simulink library "discreteClampingPID"  (R2022a)
settings: Solver=VariableStepAuto  StartTime=0.0  StopTime=10.0  RelTol=1e-3
undefined symbols (not defined in the file): Ts
libraries: simulink x4
settings Model: Creator=adabney  LastModifiedBy=maull

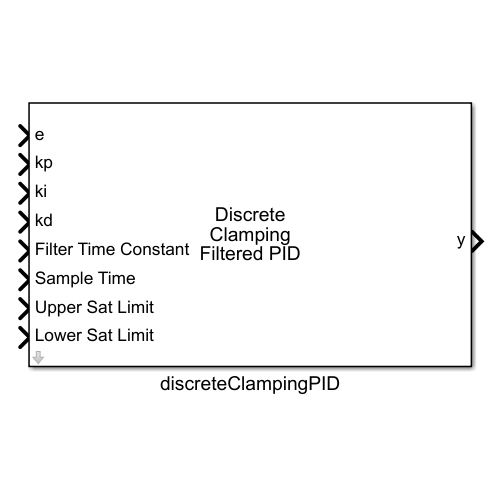
[thumbnail: Simulink's stored preview of the top-level diagram]
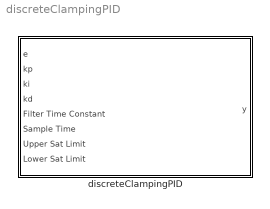
== system discreteClampingPID ==
  discreteClampingPID : Subsystem  mask{kP=1, kI=1, kD=1, tau=1, Ts=Ts, upperLim=0, lowerLim=0}
      mask prompts: kP "Proportional Gain"; kI "Integral Gain"; kD "Derivative Gain"; tau "Filter Time Constant"; Ts "Sample Time"; upperLim "Upper Limit"; lowerLim "Lower Limit"
      mask DialogControl DescTextVar Prompt: Discrete-time Filtered-PID Controller with Integral Clamping. When controller saturates, error signal feeding the integral is turned to zero to prevent integral wind up.
      mask DialogControl ParameterGroupVar Prompt: Controller Inputs
      mask DialogControl Container2 Prompt: Saturation Limits
      mask Display: disp('Discrete\nClamping\nFiltered PID');

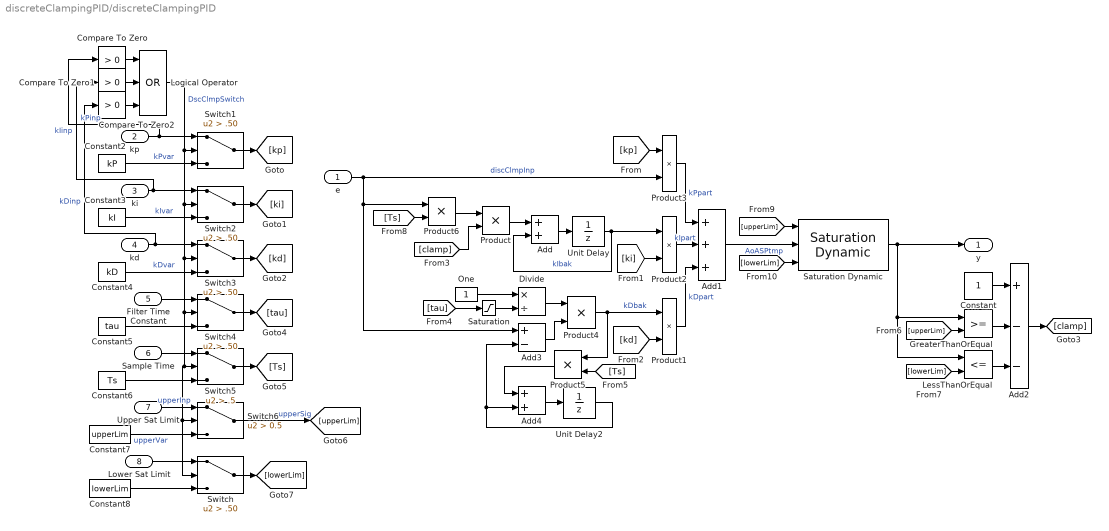
== system discreteClampingPID/discreteClampingPID ==
  e : Inport
  kp : Inport  Port=2
  ki : Inport  Port=3
  kd : Inport  Port=4
  Filter Time Constant : Inport  Port=5
  Sample Time : Inport  Port=6
  Upper Sat Limit : Inport  Port=7
  Lower Sat Limit : Inport  Port=8
  Add : Sum
  Add1 : Sum  Inputs=+++
  Add2 : Sum  Inputs=+--
  Add3 : Sum  Inputs=+-
  Add4 : Sum
  Compare To Zero : simulink/Logic and Bit Operations/Compare To Zero  relop=>  OutDataTypeStr=boolean
  Compare To Zero1 : simulink/Logic and Bit Operations/Compare To Zero  relop=>  OutDataTypeStr=boolean
  Compare To Zero2 : simulink/Logic and Bit Operations/Compare To Zero  relop=>  OutDataTypeStr=boolean
  Constant : Constant
  Constant2 : Constant  Value=kP
  Constant3 : Constant  Value=kI
  Constant4 : Constant  Value=kD
  Constant5 : Constant  Value=tau
  Constant6 : Constant  Value=Ts
  Constant7 : Constant  Value=upperLim
  Constant8 : Constant  Value=lowerLim
  Divide : Product  Inputs=*/
  GreaterThanOrEqual : RelationalOperator  OutDataTypeStr=boolean  RndMeth=Simplest  InputSameDT=off
  LessThanOrEqual : RelationalOperator  Operator=<=  OutDataTypeStr=boolean  RndMeth=Simplest  InputSameDT=off
  Logical Operator : Logic  Operator=OR  Inputs=3  AllPortsSameDT=off  OutDataTypeStr=boolean
  One : Constant  OutDataTypeStr=Inherit: Inherit via back propagation
  Product{,1..6} (7 alike) : Product
  Saturation : Saturate  UpperLimit=1000  LowerLimit=0.02
  Saturation Dynamic : simulink/Discontinuities/Saturation Dynamic  OutMin=[]  OutMax=[]  OutDataTypeStr=Inherit: Same as second input  OutDataType=fixdt(1, 16)  OutScaling=2^-10  DoSatur=off
  Switch{,1..4} (5 alike) : Switch  Criteria=u2 > Threshold  Threshold=.50  SaturateOnIntegerOverflow=off  InputSameDT=off
  Switch5 : Switch  Criteria=u2 > Threshold  Threshold=.5  SaturateOnIntegerOverflow=off  InputSameDT=off
  Switch6 : Switch  Criteria=u2 > Threshold  Threshold=0.5  SaturateOnIntegerOverflow=off  InputSameDT=off
  Unit Delay : UnitDelay  SampleTime=-1  HasFrameUpgradeWarning=on
  Unit Delay2 : UnitDelay  SampleTime=-1  HasFrameUpgradeWarning=on
  y : Outport
  wires:
  Product1/1 -> Add1/3  "kDpart"
  Product3/1 -> Add1/1  "kPpart"
  e/1 -> Product3/2, Add3/1, Product6/1  "discClmpInp"
  [kd] -> Product1/2
  [ki] -> Product2/2
  [kp] -> Product3/1
  Add1/1 -> Saturation Dynamic/2  "AoASPtmp"
  Product2/1 -> Add1/2  "kIpart"
  Add3/1 -> Product4/2
  Saturation Dynamic/1 -> y/1, GreaterThanOrEqual/1, LessThanOrEqual/1
  LessThanOrEqual/1 -> Add2/3
  GreaterThanOrEqual/1 -> Add2/2
  Constant/1 -> Add2/1
  Add/1 -> Unit Delay/1
  Product6/1 -> Product/1
  [clamp] -> Product/2
  Product/1 -> Add/1
  Add2/1 -> [clamp]
  Product4/1 -> Product1/1, Product5/1  "kDbak"
  Add4/1 -> Unit Delay2/1
  Product5/1 -> Add4/1
  Unit Delay/1 -> Product2/1, Add/2  "kIbak"
  Unit Delay2/1 -> Add4/2, Add3/2
  Divide/1 -> Product4/1
  One/1 -> Divide/1
  [Ts] -> Product5/2
  [upperLim] -> GreaterThanOrEqual/2
  [lowerLim] -> LessThanOrEqual/2
  [Ts] -> Product6/2
  [upperLim] -> Saturation Dynamic/1
  [lowerLim] -> Saturation Dynamic/3
  Switch1/1 -> [kp]
  kp/1 -> Compare To Zero/1, Switch1/1  "kPinp"
  Constant2/1 -> Switch1/3  "kPvar"
  Switch2/1 -> [ki]
  Constant3/1 -> Switch2/3  "kIvar"
  ki/1 -> Switch2/1, Compare To Zero1/1  "kIinp"
  kd/1 -> Switch3/1, Compare To Zero2/1  "kDinp"
  Constant4/1 -> Switch3/3  "kDvar"
  Switch3/1 -> [kd]
  Constant5/1 -> Switch4/3
  Switch4/1 -> [tau]
  Filter Time Constant/1 -> Switch4/1
  Sample Time/1 -> Switch5/1
  Switch5/1 -> [Ts]
  Constant6/1 -> Switch5/3
  Switch6/1 -> [upperLim]  "upperSig"
  Switch/1 -> [lowerLim]
  Upper Sat Limit/1 -> Switch6/1  "upperInp"
  Constant7/1 -> Switch6/3  "upperVar"
  Constant8/1 -> Switch/3
  Saturation/1 -> Divide/2
  [tau] -> Saturation/1
  Lower Sat Limit/1 -> Switch/1
  Compare To Zero/1 -> Logical Operator/1
  Compare To Zero1/1 -> Logical Operator/2
  Compare To Zero2/1 -> Logical Operator/3
  Logical Operator/1 -> Switch2/2, Switch3/2, Switch4/2, Switch5/2, Switch6/2, Switch/2, Switch1/2  "DscClmpSwitch"
